simulink model "VehRT_211219"  (R2019b)
settings: Solver=ode5  StartTime=0.0  StopTime=Inf  FixedStep=Ts  RelTol=1e-3  EnableMultiTasking=on
InitFcn:
  | VehRT_Init_211219;
  | Ts=0.0005;
values from neighbouring files (symbols this model uses):
  damping_p = 0.113    [VehRT_Init_211219.m]
  Ff_ab_p = 0.41    [VehRT_Init_211219.m]
  Ff_c_p = 0.4    [VehRT_Init_211219.m]
  friction_enable = 1    [VehRT_Init_211219.m]
  sigma0_p = 200    [VehRT_Init_211219.m]
  sigma1_p = (200)^0.5    (= 14.1421356237)    [VehRT_Init_211219.m]
  td = 0.01    [VehRT_Init_211219.m]
  theta_sb_p = 0.03    [VehRT_Init_211219.m]
undefined symbols (not defined in the file or in its folder): C, canChannel, D, DiscIntNeverNeededParam, g, IO306, Kf, Kr, Lf, Lr, M, magnitude, sigma, trajectory_x11_, trajectory_x12_, trajectory_x13_, trajectory_x14_, trajectory_x15_, trajectory_x16_, trajectory_x17_, trajectory_x21_, trajectory_x22_, trajectory_x23_, trajectory_x24_, trajectory_x25_, trajectory_x26_, trajectory_x27_, trajectory_y11_, trajectory_y12_, trajectory_y13_, trajectory_y14_, trajectory_y15_, trajectory_y16_, trajectory_y17_, trajectory_y21_, trajectory_y22_, trajectory_y23_, trajectory_y24_, trajectory_y25_, trajectory_y26_, trajectory_y27_, zeta
libraries: canmsglib x31, speedgoatlib_IO612 x20, slrtlib x15, simulink x5, speedgoatlib_IO133 x3, xpcutilitieslib x2, canlib x2, xpcrtudplib x2, speedgoatlib_fpga x1, speedgoatlib_fpga_dio x1, autolibshared x1, speedgoatlib_fpga_quadrature x1
(part 2 of 4)

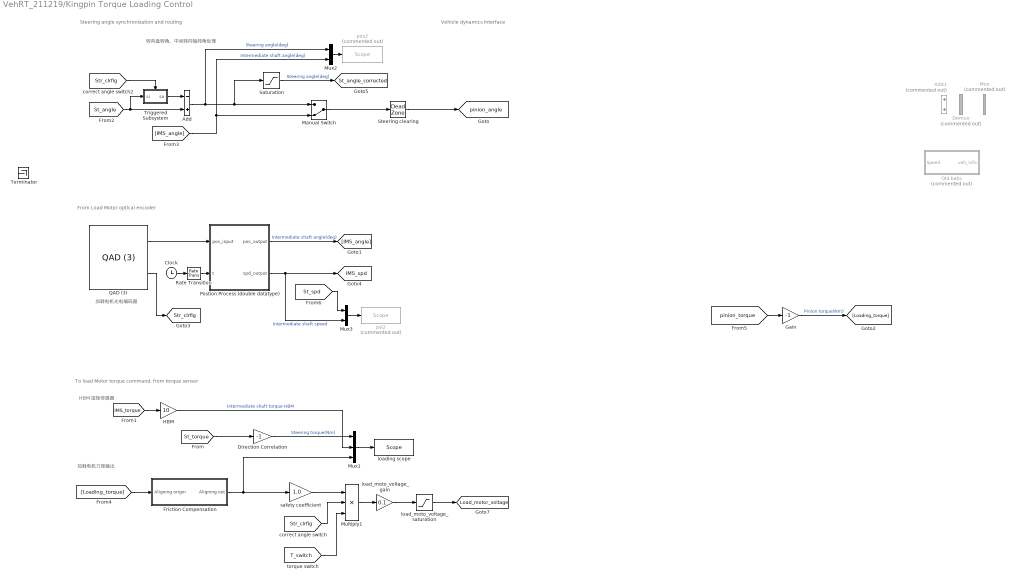
== system VehRT_211219/Kingpin Torque Loading Control ==
  note: To load Motor torque command, from torque sensor
  note: From Load Motor optical encoder
  note: Vehicle dynamics Interface
  note: Steering angle synchronization and routing
  note: 加载电机力矩输出
  note: 加载电机光电编码器
  note: HBM 扭矩传感器
  note: 转向盘转角、中间转向轴转角处理
  Add : Sum  Inputs=-+
  Add1 : Sum  Commented=on
  Clock : Clock
  Demux : Demux  Commented=on  Outputs=2
  Direction Correlation : Gain  Gain=-1
  Friction Compensation : Subsystem
  Gain : Gain  Gain=-1
  HBM : Gain  Gain=10
  Manual Switch : ManualSwitch  CurrentSetting=0
  Multiply1 : Product  Inputs=3
  Mux : Mux  Commented=on  Inputs=2
  Mux1 : Mux  Inputs=3
  Mux2 : Mux  Inputs=2
  Mux3 : Mux  Inputs=2
  Old baks : Subsystem  Commented=on
  Postion Process (double datatype) : MATLAB Function  TreatAsAtomicUnit=on
  QAD (3) : speedgoatlib_fpga_quadrature/QAD (3)  id=1  board=IO306-25k  chan=[1]  resetOnStart=on  ts=Ts  pciSlot=-1  operatingMode=Quadrature decoder  indexControlMode=Reset on index  resolution=4x  stepsPerRevolution=[6815744/2]  latchMode=Disabled  interpolatePosition=off  invertAB=off  showClearPositionInput=off  showClearIndexFoundInput=off  showPositionOutput=on  showTurnOutput=off  showSpeedOutput=off  showDirectionOutput=off  showIndexFoundOutput=on
      settings: SourceProductName=Simulink Real-Time: Speedgoat I/O Driver Library
  Rate Transition : RateTransition  Deterministic=off
  Saturation : Saturate  UpperLimit=90  LowerLimit=-90
  Steering clearing : DeadZone  LowerValue=0  UpperValue=0  SaturateOnIntegerOverflow=on
  Terminator : Terminator
  Triggered Subsystem : Subsystem  TreatAsAtomicUnit=on
  load_moto_voltage_gain : Gain  Gain=0.1
  load_moto_voltage_saturation : Saturate  UpperLimit=2.5  LowerLimit=-2.5
  loading scope : slrtlib/Displays and Logging/Scope   scopeno=3  scopetype=Target  autostart=on  viewmode=Graphical rolling  formatstr='%15.6f'  grid=on  ylimits=[-20,20]  nosamples=1000  noprepostsamples=0  interleave=1  triggermode=FreeRun  triggersignal=1  trigsignalfromport=off  triggerlevel=0.0  triggerslope=Either  triggerscope=1  triggersample=0  filename=data.dat  mode=Lazy  writesize=512  autorestart=off  dynamicfilemode=off  maxwritefilesize=512*1024^2
  "pos2 " : slrtlib/Displays and Logging/Scope   Commented=on  scopeno=1  scopetype=Target  autostart=on  viewmode=Graphical rolling  formatstr='%15.6f'  grid=on  ylimits=[-60,60]  nosamples=1000  noprepostsamples=0  interleave=1  triggermode=FreeRun  triggersignal=1  trigsignalfromport=off  triggerlevel=0.0  triggerslope=Either  triggerscope=1  triggersample=0  filename=data.dat  mode=Lazy  writesize=512  autorestart=off  dynamicfilemode=off  maxwritefilesize=512*1024^2
  psi2 : slrtlib/Displays and Logging/Scope   Commented=on  scopeno=2  scopetype=Target  autostart=on  viewmode=Graphical rolling  formatstr='%15.6f'  grid=on  ylimits=[-100,100]  nosamples=1000  noprepostsamples=0  interleave=1  triggermode=FreeRun  triggersignal=1  trigsignalfromport=off  triggerlevel=0.0  triggerslope=Either  triggerscope=1  triggersample=0  filename=data.dat  mode=Lazy  writesize=512  autorestart=off  dynamicfilemode=off  maxwritefilesize=512*1024^2
  safety coefficient : Gain  Gain=1.0
  tag scope: IMS_spd=global, Load_motor_voltage=global, St_angle_corrected=global, Str_clrflg=global, pinion_angle=global
  wires:
  load_moto_voltage_gain/1 -> load_moto_voltage_saturation/1
  HBM/1 -> Mux1/2  "Intermediate shaft torque HBM"
  Gain/1 -> [Loading_torque]  "Pinion torque(Nm)"
  [IMS_torque] -> HBM/1
  Add/1 -> Manual Switch/1, Saturation/1, Mux2/1  "Steering angle(deg)"
  QAD (3)/1 -> Postion Process (double datatype)/1(pos_input)
  [IMS_angle] -> Manual Switch/2, Mux2/2  "Intermediate shaft angle(deg)"
  Postion Process (double datatype)/1(pos_output) -> [IMS_angle]  "Intermediate shaft angle(deg)"
  safety coefficient/1 -> Multiply1/1
  load_moto_voltage_saturation/1 -> [Load_motor_voltage]
  Mux1/1 -> loading scope/1
  Manual Switch/1 -> Steering clearing/1
  Clock/1 -> Rate Transition/1
  Rate Transition/1 -> Postion Process (double datatype)/2(t)
  QAD (3)/2 -> [Str_clrflg]
  Postion Process (double datatype)/2(spd_output) -> [IMS_spd], Mux3/2  "Intermediate shaft speed"
  Triggered Subsystem/1(so) -> Add/1
  [Str_clrflg] -> Triggered Subsystem/Trigger
  [St_angle] -> Add/2, Triggered Subsystem/1(si)
  [Str_clrflg] -> Multiply1/2
  Multiply1/1 -> load_moto_voltage_gain/1
  [T_switch] -> Multiply1/3
  Mux2/1 -> "pos2 "/1
  Mux3/1 -> psi2/1
  [St_spd] -> Mux3/1
  [St_torque] -> Direction Correlation/1
  Direction Correlation/1 -> Mux1/1  "Steering torque(Nm)"
  Friction Compensation/1(Aligning out) -> safety coefficient/1, Mux1/3
  [Loading_torque] -> Friction Compensation/1(Aligning origin)
  Saturation/1 -> [St_angle_corrected]  "Steering angle(deg)"
  Steering clearing/1 -> [pinion_angle]
  [pinion_torque] -> Gain/1

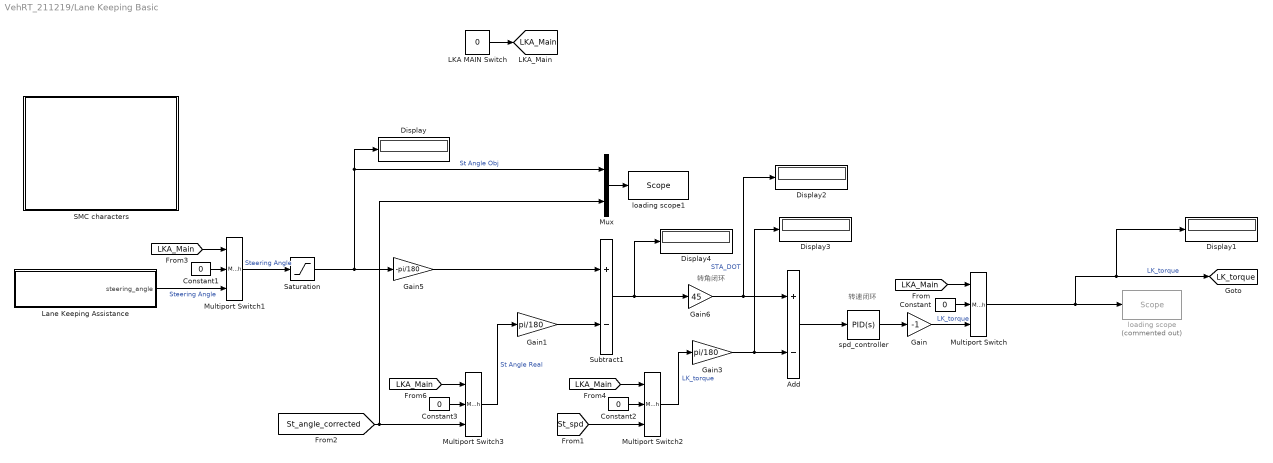
== system VehRT_211219/Lane Keeping Basic ==
  note: 转角闭环
  note: 转速闭环
  Add : Sum  Inputs=+-
  Constant{,1..3} (4 alike) : Constant  Value=0
  Display{,1..4} (5 alike) : Display
  Gain : Gain  Gain=-1
  Gain1 : Gain  Gain=pi/180
  Gain3 : Gain  Gain=pi/180
  Gain5 : Gain  Gain=-pi/180
  Gain6 : Gain  Gain=45
  LKA MAIN Switch : Constant  Value=0
  Lane Keeping Assistance : Subsystem
  Multiport Switch{,1..3} (4 alike) : MultiPortSwitch  DataPortOrder=Zero-based contiguous  Inputs=2  zeroidx=on
  Mux : Mux  Inputs=2
  SMC characters : Subsystem
  Saturation : Saturate  UpperLimit=70  LowerLimit=-70
  Subtract1 : Sum  Inputs=+-
  loading scope : slrtlib/Displays and Logging/Scope   Commented=on  scopeno=7  scopetype=Target  autostart=on  viewmode=Graphical rolling  formatstr='%15.6f'  grid=on  ylimits=[-2.5,2.5]  nosamples=1000  noprepostsamples=0  interleave=1  triggermode=FreeRun  triggersignal=1  trigsignalfromport=off  triggerlevel=0.0  triggerslope=Either  triggerscope=1  triggersample=0  filename=data.dat  mode=Lazy  writesize=512  autorestart=off  dynamicfilemode=off  maxwritefilesize=512*1024^2
  loading scope1 : slrtlib/Displays and Logging/Scope   scopeno=6  scopetype=Target  autostart=on  viewmode=Graphical rolling  formatstr='%15.6f'  grid=on  ylimits=[-50,50]  nosamples=1000  noprepostsamples=0  interleave=1  triggermode=FreeRun  triggersignal=1  trigsignalfromport=off  triggerlevel=0.0  triggerslope=Either  triggerscope=1  triggersample=0  filename=data.dat  mode=Lazy  writesize=512  autorestart=off  dynamicfilemode=off  maxwritefilesize=512*1024^2
  spd_controller : simulink/Continuous/PID Controller  Controller=PID  Form=Parallel  TimeDomain=Continuous-time  SampleTime=-1  IntegratorMethod=Forward Euler  FilterMethod=Forward Euler  ControllerParametersSource=internal  P=4.3  I=0  D=0.03  UseFilter=on  N=100  TunerSelectOption=Transfer Function Based (PID Tuner App)  InitialConditionSource=internal  InitialConditionForIntegrator=0  InitialConditionForFilter=0  DifferentiatorICPrevScaledInput=0  ExternalReset=none  TrackingMode=off  Kt=1  LimitOutput=on  UpperSaturationLimit=7  LowerSaturationLimit=-7  LinearizeAsGain=off  AntiWindupMode=none  Kb=1  POutMin=[]  POutMax=[]  IOutMin=[]  IOutMax=[]  DOutMin=[]  DOutMax=[]  NOutMin=[]  NOutMax=[]  SumOutMin=[]  SumOutMax=[]  SaturationOutMin=[]  SaturationOutMax=[]  PParamMin=[]  PParamMax=[]  IParamMin=[]  IParamMax=[]  DParamMin=[]  DParamMax=[]  NParamMin=[]  NParamMax=[]  KbParamMin=[]  KbParamMax=[]  KtParamMin=[]  KtParamMax=[]  KbOutMin=[]  KbOutMax=[]  KtOutMin=[]  KtOutMax=[]  IntegratorOutMin=[]  IntegratorOutMax=[]  FilterOutMin=[]  FilterOutMax=[]  SumI1OutMin=[]  SumI1OutMax=[]  SumI2OutMin=[]  SumI2OutMax=[]  SumI3OutMin=[]  SumI3OutMax=[]  SumI4OutMin=[]  SumI4OutMax=[]  SumDOutMin=[]  SumDOutMax=[]  DifferentiatorOutMin=[]  DifferentiatorOutMax=[]  FilterDiffOutCoefMin=[]  FilterDiffOutCoefMax=[]  ReciprocalOutMin=[]  ReciprocalOutMax=[]  SumDenOutMin=[]  SumDenOutMax=[]  SumNumOutMin=[]  SumNumOutMax=[]  DivideOutMin=[]  DivideOutMax=[]  IntegratorContinuousStateAttributes=''  IntegratorStateMustResolveToSignalObject=off  IntegratorRTWStateStorageClass=Auto  FilterContinuousStateAttributes=''  FilterStateMustResolveToSignalObject=off  FilterRTWStateStorageClass=Auto  ParallelPVariant=InternalParameters  IdealPVariant=Disabled  IVariant=InternalParameters  DVariant=InternalParameters  IntegratorVariant=Continuous  SatVariant=Enabled  AWVariant=Passthrough  PCopyVariant=Disabled  TRVariant=Disabled  FdbkBlocksVariant=Forward  IdealPFdbkVariant=Disabled  SatFdbkVariant=Disabled  DerivativeFilterVariant=ContFilter  NVariant=InternalParameters  NCopyVariant=Disabled  FilterICVariant=InternalICsFilter  IntegratorICVariant=InternalICs  ExternalResetVariant=Disabled  TRSumVariant=Passthrough  SumFdbkVariant=Disabled  SumVariant=Sum_PID
  tag scope: LKA_Main=global, LK_torque=global
  wires:
  Subtract1/1 -> Gain6/1, Display4/1
  Multiport Switch3/1 -> Gain1/1  "St Angle Real"
  Gain1/1 -> Subtract1/2
  Gain6/1 -> Display2/1, Add/1  "STA_DOT"
  Multiport Switch/1 -> loading scope/1, Display1/1, [LK_torque]  "LK_torque"
  [St_spd] -> Multiport Switch2/3
  Gain3/1 -> Display3/1, Add/2
  Add/1 -> spd_controller/1
  Mux/1 -> loading scope1/1
  spd_controller/1 -> Gain/1
  Saturation/1 -> Gain5/1, Mux/1, Display/1  "St Angle Obj"
  Multiport Switch1/1 -> Saturation/1  "Steering Angle"
  Gain5/1 -> Subtract1/1
  LKA MAIN Switch/1 -> [LKA_Main]
  [LKA_Main] -> Multiport Switch/1
  Constant/1 -> Multiport Switch/2
  Gain/1 -> Multiport Switch/3  "LK_torque"
  Constant1/1 -> Multiport Switch1/2
  [LKA_Main] -> Multiport Switch1/1
  Lane Keeping Assistance/1(steering_angle) -> Multiport Switch1/3  "Steering Angle"
  Constant2/1 -> Multiport Switch2/2
  [LKA_Main] -> Multiport Switch2/1
  Multiport Switch2/1 -> Gain3/1  "LK_torque"
  [LKA_Main] -> Multiport Switch3/1
  Constant3/1 -> Multiport Switch3/2
  [St_angle_corrected] -> Multiport Switch3/3, Mux/2

== system VehRT_211219/Vehicle Info ==
  Bus Selector : BusSelector  OutputSignals=drv_sta,drv_thr,drv_brk
  "Scope " : slrtlib/Displays and Logging/Scope   scopeno=112  scopetype=Target  autostart=on  viewmode=Graphical rolling  formatstr='%15.6f'  grid=on  ylimits=[0,1]  nosamples=8000  noprepostsamples=0  interleave=1  triggermode=FreeRun  triggersignal=1  trigsignalfromport=off  triggerlevel=0.0  triggerslope=Either  triggerscope=1  triggersample=0  filename=data.dat  mode=Lazy  writesize=512  autorestart=off  dynamicfilemode=off  maxwritefilesize=512*1024^2
  Scope 1 : slrtlib/Displays and Logging/Scope   scopeno=113  scopetype=Target  autostart=on  viewmode=Graphical rolling  formatstr='%15.6f'  grid=on  ylimits=[0,1]  nosamples=8000  noprepostsamples=0  interleave=1  triggermode=FreeRun  triggersignal=1  trigsignalfromport=off  triggerlevel=0.0  triggerslope=Either  triggerscope=1  triggersample=0  filename=data.dat  mode=Lazy  writesize=512  autorestart=off  dynamicfilemode=off  maxwritefilesize=512*1024^2
  Scope 2 : slrtlib/Displays and Logging/Scope   scopeno=111  scopetype=Target  autostart=on  viewmode=Graphical rolling  formatstr='%15.6f'  grid=on  ylimits=[-60,60]  nosamples=8000  noprepostsamples=0  interleave=1  triggermode=FreeRun  triggersignal=1  trigsignalfromport=off  triggerlevel=0.0  triggerslope=Either  triggerscope=1  triggersample=0  filename=data.dat  mode=Lazy  writesize=512  autorestart=off  dynamicfilemode=off  maxwritefilesize=512*1024^2
  drv_brk : Gain
  drv_sta : Gain
  drv_thr : Gain
  wires:
  [Veh_info] -> Bus Selector/1
  Bus Selector/1 -> drv_sta/1  "<drv_sta>"
  Bus Selector/2 -> drv_thr/1  "<drv_thr>"
  Bus Selector/3 -> drv_brk/1  "<drv_brk>"
  drv_thr/1 -> "Scope "/1  "drv_thr"
  drv_brk/1 -> Scope 1/1  "drv_brk"
  drv_sta/1 -> Scope 2/1  "drv_sta"

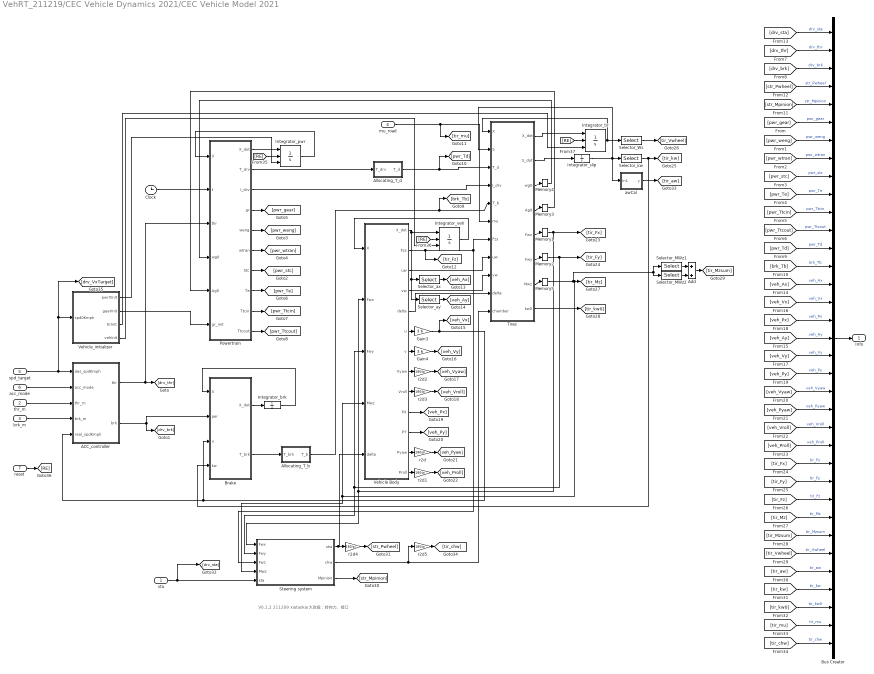
== system VehRT_211219/CEC Vehicle Dynamics 2021/CEC Vehicle Model 2021 ==
  note: V0.1.2 211209 xiataokai 大改版：转向力、接口
  sta : Inport
  thr_m : Inport  Port=2
  brk_m : Inport  Port=3
  mu_road : Inport  Port=4
  spd_target : Inport  Port=5
  acc_mode : Inport  Port=6
  reset : Inport  Port=7
  ACC_controller : Subsystem
  Add : Sum
  Allocating_T_b : Subsystem
  Allocating_T_d : Subsystem
  Brake : MATLAB Function
  Bus Creator : BusCreator  Inputs=35
  Clock : Clock
  Gain3 : Gain  Gain=3.6
  Gain4 : Gain  Gain=3.6
  Integrator_brk : Integrator  InitialCondition=zeros(5,1)  LimitOutput=on  UpperSaturationLimit=[1e9;1e9;1e9;1e9;1e9]  LowerSaturationLimit=[-1e9;-1e9;-1e9;-1e9;-1e9]
  Integrator_pwr : Integrator  ExternalReset=rising  InitialConditionSource=external  InitialCondition=[750/60*2*pi;0;0]  LimitOutput=on  UpperSaturationLimit=[1e9;1e9;1e9]  LowerSaturationLimit=[-1e9;-1e9;-1e9]
  Integrator_slip : Integrator  InitialCondition=zeros(8,1)  LimitOutput=on  UpperSaturationLimit=[1e9;1e9;1e9;1e9;1e9;1e9;1e9;1e9]  LowerSaturationLimit=[-1e9;-1e9;-1e9;-1e9;-1e9;-1e9;-1e9;-1e9]
  Integrator_tir : Integrator  ExternalReset=rising  InitialConditionSource=external  InitialCondition=zeros(6,1)  LimitOutput=on  UpperSaturationLimit=[1e9;1e9;1e9;1e9;1e9;1e9]  LowerSaturationLimit=[0;0;0;0;-1e9;-1e9]
  Integrator_veh : Integrator  ExternalReset=rising  InitialConditionSource=external  InitialCondition=zeros(8,1)  LimitOutput=on  UpperSaturationLimit=[1e9;1e9;1e9;1e9;1e9;1e9;1e9;1e9]  LowerSaturationLimit=[-1e9;-1e9; 0;-1e9;-1e9;-1e9;-1e9;-1e9]
  Memory{1..5} (5 alike) : Memory
  Powertrain : MATLAB Function
  Selector_MWz1 : Selector  InputPortWidth=4  IndexOptions=Index vector (dialog)  Indices=[1]  OutputSizes=1
  Selector_MWz2 : Selector  InputPortWidth=4  IndexOptions=Index vector (dialog)  Indices=[2]  OutputSizes=1
  Selector_Ws : Selector  InputPortWidth=6  IndexOptions=Index vector (dialog)  Indices=[1:4]  OutputSizes=1
  Selector_ax : Selector  InputPortWidth=8  IndexOptions=Index vector (dialog)  Indices=[3]  OutputSizes=1
  Selector_ay : Selector  InputPortWidth=8  IndexOptions=Index vector (dialog)  Indices=[4]  OutputSizes=1
  Selector_kw : Selector  InputPortWidth=8  IndexOptions=Index vector (dialog)  Indices=[1:4]  OutputSizes=1
  Steering system : Subsystem
  Tires : MATLAB Function  SystemSampleTime=0.001
  Vehicle Body : MATLAB Function  TreatAsAtomicUnit=on
      settings: MinAlgLoopOccurrences=on
  Vehicle_initializer : Subsystem
  awCal : Subsystem
  r2d{,1..5} (6 alike) : Gain  Gain=180/pi
  Info : Outport  VectorParamsAs1DForOutWhenUnconnected=off
  wires:
  Vehicle Body/12(Pyaw) -> r2d/1
  Vehicle_initializer/2(gearInit) -> Powertrain/6(gr_init)
  Tires/7(Mwz) -> Memory5/1
  Vehicle_initializer/1(pwrXInit) -> Integrator_pwr/3
  Vehicle_initializer/4(vehInit) -> Integrator_veh/3
  Memory2/1 -> [tir_Fy], Steering system/2(Fwy), Vehicle Body/3(Fwy)
  Powertrain/7(Stc) -> [pwr_stc]
  [RE] -> Integrator_veh/2
  [RE] -> Integrator_tir/2
  spd_target/1 -> [drv_VxTarget], Vehicle_initializer/1(spd0Kmph), ACC_controller/1(des_spdKmph)
  Selector_ax/1 -> [veh_Ax]
  Add/1 -> [tir_Mzsum]
  Clock/1 -> Powertrain/2(t)
  Integrator_pwr/1 -> Powertrain/1(X)
  Vehicle Body/4(vw) -> Tires/9(vw)
  Integrator_brk/1 -> Brake/1(X)
  Powertrain/2(T_drv) -> Allocating_T_d/1(T_drv)
  Gain3/1 -> [veh_Vx], ACC_controller/5(real_spdKmph), Brake/3(u)
  Brake/1(X_dot) -> Integrator_brk/1
  Brake/2(T_brk) -> Allocating_T_b/1(T_brk)
  Tires/6(Fwy) -> Memory2/1
  r2d3/1 -> [veh_Vroll]
  Gain4/1 -> [veh_Vy]
  Powertrain/6(wtran) -> [pwr_wtran]
  r2d2/1 -> [veh_Vyaw]
  Vehicle Body/6(u) -> Gain3/1
  Powertrain/5(weng) -> [pwr_weng]
  Allocating_T_d/1(T_d) -> [pwr_Td], Tires/3(T_d)
  ACC_controller/1(thr) -> Powertrain/3(thr), [drv_thr]
  Tires/2(S_dot) -> Integrator_slip/1
  Vehicle Body/3(uw) -> Tires/8(uw)
  [RE] -> Integrator_pwr/2
  Integrator_veh/1 -> Vehicle Body/1(X)
  Selector_ay/1 -> [veh_Ay]
  Vehicle Body/7(v) -> Gain4/1
  Tires/5(Fwx) -> Memory1/1
  Powertrain/3(I_drv) -> Tires/4(I_drv)
  Memory3/1 -> Powertrain/5(Ag0)
  Vehicle Body/5(delta) -> Tires/10(delta)
  Selector_MWz2/1 -> Add/2
  Powertrain/1(X_dot) -> Integrator_pwr/1
  mu_road/1 -> [tir_mu], Tires/6(mu)
  r2d1/1 -> [veh_Proll]
  Tires/3(wg0) -> Memory4/1
  Tires/4(Ag0) -> Memory3/1
  Selector_MWz1/1 -> Add/1
  ACC_controller/2(brk) -> Brake/2(per), [drv_brk]
  Vehicle Body/8(Vyaw) -> r2d2/1
  Integrator_slip/1 -> awCal/1(In1), Tires/2(S), Selector_kw/1
  Powertrain/4(gr) -> [pwr_gear]
  Selector_Ws/1 -> [tir_Vwheel]
  Integrator_tir/1 -> Tires/1(X), Selector_Ws/1
  Vehicle_initializer/3(tirInit) -> Integrator_tir/3
  Vehicle Body/9(Vroll) -> r2d3/1
  Vehicle Body/13(Proll) -> r2d1/1
  Memory4/1 -> Powertrain/4(wg0)
  Vehicle Body/1(X_dot) -> Selector_ax/1, Selector_ay/1, Integrator_veh/1
  Memory1/1 -> [tir_Fx], Steering system/1(Fwx), Vehicle Body/2(Fwx)
  Vehicle Body/2(Fzs) -> [tir_Fz], Steering system/3(Fwz), Tires/7(Fzs)
  Allocating_T_b/1(T_b) -> [brk_Tb], Tires/5(T_b)
  Selector_kw/1 -> [tir_kw], Brake/4(kw)
  Tires/1(X_dot) -> Integrator_tir/1
  r2d/1 -> [veh_Pyaw]
  Tires/8(kw0) -> [tir_kw0]
  Memory5/1 -> [tir_Mz], Steering system/4(Mwz), Vehicle Body/4(Mwz), Selector_MWz2/1, Selector_MWz1/1
  sta/1 -> [drv_sta], Steering system/5(sta)
  Steering system/1(stw) -> Vehicle Body/5("delta "), r2d4/1
  Steering system/3(Mpinion) -> [str_Mpinion]
  Steering system/2(chw) -> Tires/11(chamber), r2d5/1
  Vehicle Body/10(PX) -> [veh_Px]
  Vehicle Body/11(PY) -> [veh_Py]
  Powertrain/8(Te) -> [pwr_Te]
  Powertrain/9(Ttcin) -> [pwr_Ttcin]
  Powertrain/10(Ttcout) -> [pwr_Ttcout]
  r2d4/1 -> [str_Pwheel]
  awCal/1(y) -> [tir_aw]
  [drv_sta] -> Bus Creator/1  "drv_sta"
  [drv_thr] -> Bus Creator/2  "drv_thr"
  [drv_brk] -> Bus Creator/3  "drv_brk"
  [str_Pwheel] -> Bus Creator/4  "str_Pwheel"
  [str_Mpinion] -> Bus Creator/5  "str_Mpinion"
  [pwr_gear] -> Bus Creator/6  "pwr_gear"
  [pwr_weng] -> Bus Creator/7  "pwr_weng"
  [pwr_wtran] -> Bus Creator/8  "pwr_wtran"
  [pwr_stc] -> Bus Creator/9  "pwr_stc"
  [pwr_Te] -> Bus Creator/10  "pwr_Te"
  [pwr_Ttcin] -> Bus Creator/11  "pwr_Ttcin"
  [pwr_Ttcout] -> Bus Creator/12  "pwr_Ttcout"
  [pwr_Td] -> Bus Creator/13  "pwr_Td"
  [brk_Tb] -> Bus Creator/14  "brk_Tb"
  [veh_Ax] -> Bus Creator/15  "veh_Ax"
  [veh_Vx] -> Bus Creator/16  "veh_Vx"
  [veh_Px] -> Bus Creator/17  "veh_Px"
  [veh_Ay] -> Bus Creator/18  "veh_Ay"
  [veh_Vy] -> Bus Creator/19  "veh_Vy"
  [veh_Py] -> Bus Creator/20  "veh_Py"
  [veh_Vyaw] -> Bus Creator/21  "veh_Vyaw"
  [veh_Pyaw] -> Bus Creator/22  "veh_Pyaw"
  [veh_Vroll] -> Bus Creator/23  "veh_Vroll"
  [veh_Proll] -> Bus Creator/24  "veh_Proll"
  [tir_Fx] -> Bus Creator/25  "tir_Fx"
  [tir_Fy] -> Bus Creator/26  "tir_Fy"
  [tir_Fz] -> Bus Creator/27  "tir_Fz"
  [tir_Mz] -> Bus Creator/28  "tir_Mz"
  [tir_Mzsum] -> Bus Creator/29  "tir_Mzsum"
  [tir_Vwheel] -> Bus Creator/30  "tir_Vwheel"
  [tir_aw] -> Bus Creator/31  "tir_aw"
  [tir_kw] -> Bus Creator/32  "tir_kw"
  [tir_kw0] -> Bus Creator/33  "tir_kw0"
  [tir_mu] -> Bus Creator/34  "tir_mu"
  [tir_chw] -> Bus Creator/35  "tir_chw"
  r2d5/1 -> [tir_chw]
  Bus Creator/1 -> Info/1
  acc_mode/1 -> ACC_controller/2(acc_mode)
  thr_m/1 -> ACC_controller/3(thr_m)
  brk_m/1 -> ACC_controller/4(brk_m)
  reset/1 -> [RE]

== system VehRT_211219/CEC Vehicle Dynamics 2021/Reset with Clutch ==
  Clock : Clock
  Reset Funvtion : MATLAB Function  TreatAsAtomicUnit=on  SystemSampleTime=0.001
  rst : Outport
  wires:
  Reset Funvtion/1(rst) -> rst/1
  Clock/1 -> Reset Funvtion/2(t)
  [pedal_clt] -> Reset Funvtion/1(clt)

== system VehRT_211219/CEC Vehicle Dynamics 2021/mu_test ==
  Manual Switch : ManualSwitch  CurrentSetting=0
  Vector Concatenate : Concatenate  NumInputs=4
  mu=0.85 : Constant  Value=ones(4,1)*0.85
  mu=1~0.2 : Step  Time=17.5  Before=1  After=0.2  SampleTime=0
  mu=1~0.2_2 : Step  Time=17.5  Before=1  After=0.2  SampleTime=0
  mu=1~0.2_3 : Step  Time=17.5  Before=1  After=0.2  SampleTime=0
  mu=1~0.2_4 : Step  Time=17.5  Before=1  After=0.2  SampleTime=0
  mus : Outport
  wires:
  mu=1~0.2_4/1 -> Vector Concatenate/4
  mu=1~0.2/1 -> Vector Concatenate/1
  mu=1~0.2_2/1 -> Vector Concatenate/2
  Vector Concatenate/1 -> Manual Switch/1
  mu=1~0.2_3/1 -> Vector Concatenate/3
  Manual Switch/1 -> mus/1
  mu=0.85/1 -> Manual Switch/2

== system VehRT_211219/Connect Scenery/Backup ==
  "Byte Packing " : xpcutilitieslib/Byte Packing   Commented=on  MaskPackedDataType=uint8  MaskUnpackedDataTypes={'double'}  MaskAlignment=1
  Byte Unpacking 1 : xpcutilitieslib/Byte Unpacking   Commented=on  MaskUnpackedDataTypes={'double'}  MaskUnpackedDataSizes={[2]}  MaskAlignment=1
      settings: SourceProductName=Simulink Real-Time  SourceProductBaseCode=XP
  CAN Configuration : canlib/CAN Configuration  Commented=on  BlockHandle=1343.0002  Device=MathWorks Virtual 1 (Channel 1)  DeviceMenu=MathWorks Virtual 1 (Channel 1)  ObjConstructor=canChannel('MathWorks', 'Virtual 1', 1)  BusSpeed=1000000  EnableBitParameters=off  SJW=1  TSEG1=4  TSEG2=3  NSamples=1  AckMode=Normal
      settings: SourceProductName=Vehicle Network Toolbox  SourceProductBaseCode=VN
  CAN Receive : canlib/CAN Receive  Commented=on  BlockHandle=1344.0002  Device=MathWorks Virtual 1 (Channel 1)  DeviceMenu=MathWorks Virtual 1 (Channel 1)  ObjConstructor=canChannel('MathWorks', 'Virtual 1', 1)  EnableStandardIDsFilter=off  StdIDsCombo=Allow all  StandardIDs=0  EnableExtendedIDsFilter=off  ExtIDsCombo=Allow all  ExtendedIDs=0  SampleTime=0.01  MsgsPerTimestep=all  InternalFilterUpdateStatus=on  BusOutput=off
      settings: SourceProductName=Vehicle Network Toolbox  SourceProductBaseCode=VN
  CAN Unpack : canmsglib/CAN Unpack  Commented=on  MsgList=(none)  MsgName=CAN Msg  MsgIDType=Standard (11-bit identifier)  MsgIdentifier=0  MsgLength=8  SignalInfo={}  IDPort=off  TimestampPort=off  ErrorPort=off  RemotePort=off  LengthPort=off  StatusPort=off  ApplyMinMax=off
      settings: SourceProductName=Vehicle Network Toolbox  SourceProductBaseCode=VN  DataFormat=raw data
  CAN Write{1..6} (6 alike) : speedgoatlib_IO612/CAN Write  id=1  sampleTime=0.005  portSelection=2  messageType=CAN  enaStatusPort=off  protl=IO612  ptIdx=1  isFDMod=0
      settings: SourceProductName=Simulink Real-Time: Speedgoat Library
  Demux1 : Demux  Commented=on  Outputs=2
  Display1 : Display  Commented=on
  From1 : From  Commented=on  GotoTag=pedal_acc  TagVisibility=global
  From4 : From  Commented=on  GotoTag=pedal_brk  TagVisibility=global
  Mux : Mux  Commented=on  Inputs=12
  Mux1 : Mux  Commented=on  Inputs=2
  Receive1 : xpcrtudplib/UDP Receive  Commented=on  ipAddressVal=Use host-target connection  localPort=22222  rcvWidth=16  rcvFmAny=off  fmAddress=192.168.7.23  rcvMulticast=off  multicastAddress=[]  maxUDPQueue=8  sampleTime=-1
      settings: SourceProductName=Simulink Real-Time
  Reference : Sin  Commented=on  SampleTime=0
  Reference2 : simulink/Sources/Repeating Sequence  Commented=on  rep_seq_t=[0 2]  rep_seq_y=[-2 2]
  Scope : Scope  Commented=on
  "Scope " : slrtlib/Displays and Logging/Scope   Commented=on  scopeno=1  scopetype=Target  autostart=on  viewmode=Graphical sliding  formatstr='%15.6f'  grid=on  ylimits=[-1,1]  nosamples=4000  noprepostsamples=0  interleave=1  triggermode=FreeRun  triggersignal=1  trigsignalfromport=off  triggerlevel=0.0  triggerslope=Either  triggerscope=1  triggersample=0  filename=data.dat  mode=Lazy  writesize=512  autorestart=off  dynamicfilemode=off  maxwritefilesize=512*1024^2
  Send1 : xpcrtudplib/UDP Send  Commented=on  ipAddressVal=Use host-target connection  localPort=-1  toAddress=192.168.7.23  toPort=1234  sampleTime=0.05
      settings: SourceProductName=Simulink Real-Time  SourceProductBaseCode=XP
  "Vxzb0 " : Gain  Commented=on
  Width : Width  Commented=on
  phi_Gain : Gain
  theta_Gain : Gain
  wires:
  ? -> Mux/11
  ? -> Mux/12
  Receive1/1 -> Byte Unpacking 1/1
  Mux/1 -> "Byte Packing "/1
  "Vxzb0 "/1 -> Scope/1
  From1/1 -> Mux/9
  Demux1/1 -> Mux1/2  "feedback"
  Byte Unpacking 1/1 -> Demux1/1  "feedback"
  Demux1/2 -> "Vxzb0 "/1
  Mux1/1 -> "Scope "/1
  Receive1/2 -> Display1/1
  Reference2/1 -> Mux/7, Mux1/1  "origin"
  "Byte Packing "/1 -> Width/1, Send1/1
  Width/1 -> Send1/2
  From4/1 -> Mux/10
  ? -> phi_Gain/1  "<phi>"
  ? -> theta_Gain/1  "<theta>"

== system VehRT_211219/Connect Scenery/CAN Receiver Port4 ==
  CAN Read1 : speedgoatlib_IO612/CAN Read  id=1  sampleTime=-1  portSelection=2  messageType=CAN  protl=IO612  ptIdx=1  isFDMod=0
      settings: SourceProductName=Simulink Real-Time: Speedgoat Library
  CAN Unpack : canmsglib/CAN Unpack  CANdbFile=D:\Speedgoat\Simulink Test Model\EPS_Test_2018_0101.dbc  MsgList=EPS2MAB  MsgName=CAN Msg  MsgIDType=Standard (11-bit identifier)  MsgIdentifier=500  MsgLength=8  SignalInfo={ 'Vx_des', '16', '32', 'LE', 'single', 'Standard', '0', '1', '0', '-Inf', 'Inf'; 'detection', '48', '16', 'LE', 'unsigned', 'Standard', '0', '1', '0', '-Inf', 'Inf'; 'road_id', '0', '16', 'LE', 'unsigned', 'Standard', '0', '1', '0', '-Inf', 'Inf' }  IDPort=off  TimestampPort=off  ErrorPort=off  RemotePort=off  LengthPort=off  StatusPort=off  ApplyMinMax=off
      settings: SourceProductName=Simulink Real-Time
  CAN Unpack1 : canmsglib/CAN Unpack  CANdbFile=D:\Speedgoat\Simulink Test Model\EPS_Test_2018_0101.dbc  MsgList=EPS2MAB  MsgName=VSS1  MsgIDType=Standard (11-bit identifier)  MsgIdentifier=501  MsgLength=8  SignalInfo={ 'range', '0', '64', 'LE', 'double', 'Standard', '0', '1', '0', '-Inf', 'Inf' }  IDPort=off  TimestampPort=off  ErrorPort=off  RemotePort=off  LengthPort=off  StatusPort=off  ApplyMinMax=off
      settings: SourceProductName=Simulink Real-Time
  CAN Unpack2 : canmsglib/CAN Unpack  CANdbFile=D:\Speedgoat\Simulink Test Model\EPS_Test_2018_0101.dbc  MsgList=EPS2MAB  MsgName=VSS2  MsgIDType=Standard (11-bit identifier)  MsgIdentifier=502  MsgLength=8  SignalInfo={ 'theta', '0', '64', 'LE', 'double', 'Standard', '0', '1', '0', '-Inf', 'Inf' }  IDPort=off  TimestampPort=off  ErrorPort=off  RemotePort=off  LengthPort=off  StatusPort=off  ApplyMinMax=off
      settings: SourceProductName=Simulink Real-Time
  CAN Unpack3 : canmsglib/CAN Unpack  CANdbFile=D:\Speedgoat\Simulink Test Model\EPS_Test_2018_0101.dbc  MsgList=EPS2MAB  MsgName=VSS3  MsgIDType=Standard (11-bit identifier)  MsgIdentifier=503  MsgLength=8  SignalInfo={ 'head_ada', '0', '64', 'LE', 'double', 'Standard', '0', '1', '0', '-Inf', 'Inf' }  IDPort=off  TimestampPort=off  ErrorPort=off  RemotePort=off  LengthPort=off  StatusPort=off  ApplyMinMax=off
      settings: SourceProductName=Simulink Real-Time
  While Iterator : WhileIterator  WhileBlockType=do-while
  detection : Outport
  Vx_des : Outport  Port=2
  devia_from_prescan : Outport  Port=3
  qulv_from_prescan : Outport  Port=4
  head_ada : Outport  Port=5
  road_id : Outport  Port=6
  wires:
  CAN Read1/1 -> While Iterator/1
  CAN Read1/2 -> CAN Unpack3/1, CAN Unpack2/1, CAN Unpack1/1, CAN Unpack/1
  CAN Unpack/1 -> Vx_des/1  "Vx_des"
  CAN Unpack/2 -> detection/1  "detection"
  CAN Unpack/3 -> road_id/1
  CAN Unpack1/1 -> devia_from_prescan/1  "range"
  CAN Unpack2/1 -> qulv_from_prescan/1  "theta"
  CAN Unpack3/1 -> head_ada/1  "head_ada"

== system VehRT_211219/EPS Steering Torque Assist Control/Backups ==
  note: 备用的滞后-超前控制
  note: 备用的超前控制
  Lag Control1 : TransferFcn  Commented=on  Numerator=[1/2/pi/4.5 1]  Denominator=[1/2/pi/1 1]
  Lead Control : TransferFcn  Commented=on  Numerator=[1/2/pi/14 1]  Denominator=[1/2/pi/181 1]
  Lead Control1 : TransferFcn  Commented=on  Numerator=[1/2/pi/14 1]  Denominator=[1/2/pi/100 1]
  Relay : Relay  Commented=on  OnSwitchValue=10  OffSwitchValue=-10
  Terminator : Terminator
  wires:
  Lag Control1/1 -> Lead Control1/1
  [Vehicle_speed] -> Terminator/1

== system VehRT_211219/Hardware Interfaces/RPM Display ==
  Bus Selector : BusSelector  OutputSignals=pwr_weng
  MATLAB Function : MATLAB Function  TreatAsAtomicUnit=on
  Out1 : Outport
  wires:
  [Veh_info] -> Bus Selector/1
  Bus Selector/1 -> MATLAB Function/1(rpm)  "<pwr_weng>"
  MATLAB Function/1(out) -> Out1/1

== system VehRT_211219/Hardware Interfaces/Shiftting Display ==
  Bus Selector : BusSelector  OutputSignals=pwr_gear
  MATLAB Function : MATLAB Function  TreatAsAtomicUnit=on
  Out1 : Outport
  wires:
  [Veh_info] -> Bus Selector/1
  Bus Selector/1 -> MATLAB Function/1(gear)  "<pwr_gear>"
  MATLAB Function/1(out) -> Out1/1

== system VehRT_211219/Hardware Interfaces/Spd Dev ==
  In1 : Inport
  Add : Sum
  Gain : Gain  Gain=0.5
  Memory : Memory
  Transfer Fcn : TransferFcn  Numerator=[100 0]  Denominator=[1 100]
  Out1 : Outport  VectorParamsAs1DForOutWhenUnconnected=off
  wires:
  In1/1 -> Transfer Fcn/1
  Transfer Fcn/1 -> Add/2, Memory/1
  Memory/1 -> Add/1
  Add/1 -> Gain/1
  Gain/1 -> Out1/1  "Steering speed(deg/s)"

== system VehRT_211219/Hardware Interfaces/Torque Switch Interface  ==
  b_on : Inport
  b_off : Inport  Port=2
  Constant1 : Constant  Value=9.9
  Multiport Switch : MultiPortSwitch  DataPortOrder=Zero-based contiguous  Inputs=2  zeroidx=on
  Sine Wave : Sin  Amplitude=6  Frequency=9  SampleTime=0
  torque switch : MATLAB Function  TreatAsAtomicUnit=on
  Out1 : Outport  VectorParamsAs1DForOutWhenUnconnected=off
  tag scope: T_switch=global
  wires:
  torque switch/1(control) -> [T_switch], Multiport Switch/1
  b_off/1 -> torque switch/2(button_off)  "b_off"
  Constant1/1 -> Multiport Switch/3
  Sine Wave/1 -> Multiport Switch/2
  Multiport Switch/1 -> Out1/1
  b_on/1 -> torque switch/1(button_on)  "b_on"

== system VehRT_211219/Hardware Interfaces/While Iterator Subsystem ==
  Add2 : Sum  Inputs=+-
  CAN Read1 : speedgoatlib_IO612/CAN Read  id=1  sampleTime=-1  portSelection=1  messageType=CAN  protl=IO612  ptIdx=0  isFDMod=0
      settings: SourceProductName=Simulink Real-Time: Speedgoat Library
  CAN Unpack : canmsglib/CAN Unpack  CANdbFile=D:\Speedgoat\Simulink Test Model\EPS_Test_2018_0101.dbc  MsgList=EPS2MAB  MsgName=EPS2MAB  MsgIDType=Standard (11-bit identifier)  MsgIdentifier=2043  MsgLength=8  SignalInfo={'MotorAngle','24','32','BE','signed','Standard','0','0.0043945','0','-Inf','Inf';'MotorCurrent','40','16','BE','signed','Standard','0','0.01','0','-Inf','Inf';'TorqueSensor','56','16','BE','signed','Standard','0','0.001','0','-Inf','Inf'}  IDPort=off  TimestampPort=on  ErrorPort=off  RemotePort=off  LengthPort=off  StatusPort=on  ApplyMinMax=off
      settings: SourceProductName=Simulink Real-Time  DataFormat=CANdb specified signals
  Demux : Demux  Commented=on  Outputs=3
  Gain3 : Gain  Gain=1/18.5
  Memory2 : Memory  InheritSampleTime=on
  Product : Product  Commented=on
  Saturation1 : Saturate  Commented=on  UpperLimit=120  LowerLimit=-120
  State-Space1 : StateSpace  Commented=on  A=[0,1,0; 0,0,1; -10/0.003^3,-10/0.003^2,-10/0.003]  B=[0;0;10/0.003^3]  C=[1,0,0;0,1,0;0,0,1]  D=[0;0;0]  InitialCondition=0
  Step : Step  Commented=on  Time=1.5  SampleTime=0
  Terminator{2..3,6,9} (4 alike) : Terminator
  Terminator4 : Terminator  Commented=on
  Terminator5 : Terminator  Commented=on
  While Iterator : WhileIterator  WhileBlockType=do-while
  st_angle : Outport  VectorParamsAs1DForOutWhenUnconnected=off
  st_torque : Outport  Port=2  VectorParamsAs1DForOutWhenUnconnected=off
  st_current : Outport  Port=3  VectorParamsAs1DForOutWhenUnconnected=off
  wires:
  CAN Unpack/2 -> st_current/1  "motor_current"
  Demux/1 -> Terminator5/1  "angle"
  CAN Read1/1 -> While Iterator/1
  CAN Read1/2 -> CAN Unpack/1
  CAN Unpack/4 -> Add2/1, Memory2/1  "TimeStamp"
  CAN Unpack/5 -> Terminator2/1
  Demux/2 -> Product/2
  Add2/1 -> Terminator3/1  "message_interval"
  Step/1 -> Product/1
  Memory2/1 -> Add2/2
  CAN Unpack/1 -> Gain3/1  "motor_angle"
  Gain3/1 -> st_angle/1, State-Space1/1  "Steering wheel angle0"
  CAN Unpack/3 -> Terminator6/1, st_torque/1  "Steering wheel torque"
  Product/1 -> Saturation1/1
  Saturation1/1 -> Terminator9/1
  State-Space1/1 -> Demux/1
  Demux/3 -> Terminator4/1  "acceleration"

== system VehRT_211219/Hardware Interfaces/alpha_dis ==
  CAN Read1 : speedgoatlib_IO612/CAN Read  id=1  sampleTime=-1  portSelection=2  messageType=CAN  protl=IO612  ptIdx=1  isFDMod=0
      settings: SourceProductName=Simulink Real-Time: Speedgoat Library
  CAN Unpack : canmsglib/CAN Unpack  CANdbFile=D:\Speedgoat\Simulink Test Model\EPS_Test_2018_0101.dbc  MsgList=EPS2MAB  MsgName=ALPHA  MsgIDType=Standard (11-bit identifier)  MsgIdentifier=450  MsgLength=8  SignalInfo={'alpha','0','32','LE','single','Standard','0','1','0','-Inf','Inf'}  IDPort=off  TimestampPort=off  ErrorPort=off  RemotePort=off  LengthPort=off  StatusPort=off  ApplyMinMax=off
      settings: SourceProductName=Simulink Real-Time
  Data Type Conversion1 : DataTypeConversion  OutMin=0  OutMax=8  OutDataTypeStr=uint16  RndMeth=Nearest
  Gain : Gain  Gain=8.5
  Saturation : Saturate  UpperLimit=8.5  LowerLimit=0
  While Iterator : WhileIterator  WhileBlockType=do-while
  alpha : Outport  VectorParamsAs1DForOutWhenUnconnected=off
  wires:
  CAN Read1/1 -> While Iterator/1
  CAN Read1/2 -> CAN Unpack/1
  CAN Unpack/1 -> Gain/1  "alpha"
  Gain/1 -> Saturation/1
  Saturation/1 -> Data Type Conversion1/1
  Data Type Conversion1/1 -> alpha/1

== system VehRT_211219/Kingpin Torque Loading Control/Friction Compensation ==
  note: 加上以后会抖，而且不怎么影响手感，所以暂时不加了
  note: 摩擦补偿
  note: 阻尼补偿
  Aligning origin : Inport
  Add : Sum
  Add1 : Sum
  DAM Friction_p : Subsystem
  Damping coefficient : Gain  Gain=damping_p
  Dead Zone : DeadZone  LowerValue=-0.15  UpperValue=0.15  SaturateOnIntegerOverflow=on
  Deg2Rad : Gain  Gain=-pi/180
  Fricompmode : Constant
  Low Pass Filter : TransferFcn  Denominator=[1/2/pi/20 1]
  Multiport Switch : MultiPortSwitch  DataPortOrder=Zero-based contiguous  Inputs=2  zeroidx=on
  Aligning out : Outport  VectorParamsAs1DForOutWhenUnconnected=off
  wires:
  Aligning origin/1 -> Multiport Switch/2, Add/1
  [IMS_spd] -> Deg2Rad/1
  Deg2Rad/1 -> Dead Zone/1, DAM Friction_p/1(velocity)
  Damping coefficient/1 -> Add1/2
  Dead Zone/1 -> Damping coefficient/1
  Add/1 -> Multiport Switch/3  "Aligning torque(Nm)"
  Multiport Switch/1 -> Aligning out/1  "Aligning torque"
  Fricompmode/1 -> Multiport Switch/1
  Add1/1 -> Low Pass Filter/1
  DAM Friction_p/1(friction) -> Add1/1
  Low Pass Filter/1 -> Add/2

== system VehRT_211219/Kingpin Torque Loading Control/Old baks ==
  note: SIMULINK三自由度车辆模型
  Speed : Inport
  1DLT_SpdPrtc : Lookup_n-D  NumberOfTableDimensions=1  BreakpointsForDimension1=[0 3 8 200]  Table=[0 0 1 1]  InternalRulePriority=Speed  RndMeth=Simplest  InputSameDT=on
  Aligning Torque Calculator : Subsystem
  Divide1 : Product  Inputs=/*
  Gain : Gain  Gain=1/3.6
  Gain2 : Gain  Gain=pi/180
  Multiply : Product
  Multiply2 : Product
  Terminator2 : Terminator
  Terminator3 : Terminator
  Trigonometric Function1 : Trigonometry  Operator=atan
  Vehicle Body 3DOF Single Track1 : autolibshared/Vehicle Body 3DOF Single Track  trackMode=Single (bicycle)  inputMode=External longitudinal velocity  frontSteerMode=on  rearSteerMode=off  windMode=off  muMode=off  extFMode=off  extMMode=off  extXo=off  extpsio=off  extxdoto=off  extro=off  extYo=off  extTamb=off  extydoto=off  aMode=2  NF=2  NR=2  m=M  a=Lf  b=Lr  h=0.35  X_o=0  xdot_o=0  CalphaMode=off  sigmaMode=off  d=0  w=[1.4,1.4]  Cy_f=Kf*2  Cy_r=Kr*2  sigma_f=.1  sigma_r=.1  alpha_f_brk=[-.1 .1]  Cy_f_data=[-9e3 9e3]  alpha_r_brk=[-.1 .1]  Cy_r_data=[-9e3 9e3]  Y_o=0  ydot_o=0  Izz=I  psi_o=0  r_o=0  Af=0  Cd=.3  Cl=.1  Cpm=.1  beta_w=[0:0.01:0.3]  Cs=[0:0.03:0.9]  Cym=[0:0.01:0.3]  Pabs=101325  Tair=273  g=g  mu=1  xdot_tol=.01  Fznom=5000  Fxtire_sat=7e4  Fytire_sat=7e4  longOff=0  latOff=0  vertOff=0  wrapAng=off
      settings: SourceProductName=Powertrain Blockset  SourceProductBaseCode=PW
  Yaw Gain : Gain
  angle_saturation_rad1 : Saturate  UpperLimit=1.5  LowerLimit=-1.5
  veh_info : Outport  VectorParamsAs1DForOutWhenUnconnected=off
  tag scope: Veh_info=global
  wires:
  Vehicle Body 3DOF Single Track1/6 -> Aligning Torque Calculator/3(Fzf)  "Fzf"
  Aligning Torque Calculator/1(Tire Aligning Torque) -> Multiply2/1
  angle_saturation_rad1/1 -> Vehicle Body 3DOF Single Track1/1, Aligning Torque Calculator/5(Delta)
  Multiply/1 -> Gain/1
  Vehicle Body 3DOF Single Track1/4 -> Terminator2/1  "psi"
  Vehicle Body 3DOF Single Track1/5 -> Yaw Gain/1  "r"
  1DLT_SpdPrtc/1 -> Multiply2/2
  Multiply2/1 -> ?
  Speed/1 -> 1DLT_SpdPrtc/1, Multiply/1
  [Str_clrflg] -> Multiply/2
  Vehicle Body 3DOF Single Track1/2 -> Divide1/1  "xdot"
  Vehicle Body 3DOF Single Track1/1 -> [Veh_info], veh_info/1
  Trigonometric Function1/1 -> Aligning Torque Calculator/1(Beta)  "Beta"
  Vehicle Body 3DOF Single Track1/7 -> Terminator3/1
  Vehicle Body 3DOF Single Track1/3 -> Divide1/2  "ydot"
  Gain/1 -> Vehicle Body 3DOF Single Track1/2, Aligning Torque Calculator/4(speed)
  Yaw Gain/1 -> Aligning Torque Calculator/2(r)  "r"
  Gain2/1 -> angle_saturation_rad1/1
  ? -> Gain2/1
  Divide1/1 -> Trigonometric Function1/1

== system VehRT_211219/Kingpin Torque Loading Control/Triggered Subsystem ==
  si : Inport
  Trigger : TriggerPort  VariantControl=Variant
  so : Outport  VectorParamsAs1DForOutWhenUnconnected=off
  wires:
  si/1 -> so/1

== system VehRT_211219/Lane Keeping Basic/Lane Keeping Assistance ==
  Constant : Constant  Value=0
  Constant1 : Constant  Value=0
  Constant2 : Constant  Value=0
  Multiport Switch : MultiPortSwitch  DataPortOrder=Zero-based contiguous  Inputs=2  zeroidx=on
  Multiport Switch1 : MultiPortSwitch  DataPortOrder=Zero-based contiguous  Inputs=2  zeroidx=on
  Multiport Switch2 : MultiPortSwitch  DataPortOrder=Zero-based contiguous  Inputs=2  zeroidx=on
  PID Controller : simulink/Continuous/PID Controller  Controller=PID  Form=Parallel  TimeDomain=Continuous-time  SampleTime=-1  IntegratorMethod=Forward Euler  FilterMethod=Forward Euler  ControllerParametersSource=internal  P=20  I=0  D=0  UseFilter=on  N=100  TunerSelectOption=Transfer Function Based (PID Tuner App)  InitialConditionSource=internal  InitialConditionForIntegrator=0  InitialConditionForFilter=0  DifferentiatorICPrevScaledInput=0  ExternalReset=none  TrackingMode=off  Kt=1  LimitOutput=off  UpperSaturationLimit=inf  LowerSaturationLimit=-inf  LinearizeAsGain=on  AntiWindupMode=none  Kb=1  POutMin=[]  POutMax=[]  IOutMin=[]  IOutMax=[]  DOutMin=[]  DOutMax=[]  NOutMin=[]  NOutMax=[]  SumOutMin=[]  SumOutMax=[]  SaturationOutMin=[]  SaturationOutMax=[]  PParamMin=[]  PParamMax=[]  IParamMin=[]  IParamMax=[]  DParamMin=[]  DParamMax=[]  NParamMin=[]  NParamMax=[]  KbParamMin=[]  KbParamMax=[]  KtParamMin=[]  KtParamMax=[]  KbOutMin=[]  KbOutMax=[]  KtOutMin=[]  KtOutMax=[]  IntegratorOutMin=[]  IntegratorOutMax=[]  FilterOutMin=[]  FilterOutMax=[]  SumI1OutMin=[]  SumI1OutMax=[]  SumI2OutMin=[]  SumI2OutMax=[]  SumI3OutMin=[]  SumI3OutMax=[]  SumI4OutMin=[]  SumI4OutMax=[]  SumDOutMin=[]  SumDOutMax=[]  DifferentiatorOutMin=[]  DifferentiatorOutMax=[]  FilterDiffOutCoefMin=[]  FilterDiffOutCoefMax=[]  ReciprocalOutMin=[]  ReciprocalOutMax=[]  SumDenOutMin=[]  SumDenOutMax=[]  SumNumOutMin=[]  SumNumOutMax=[]  DivideOutMin=[]  DivideOutMax=[]  IntegratorContinuousStateAttributes=''  IntegratorStateMustResolveToSignalObject=off  IntegratorRTWStateStorageClass=Auto  FilterContinuousStateAttributes=''  FilterStateMustResolveToSignalObject=off  FilterRTWStateStorageClass=Auto  ParallelPVariant=InternalParameters  IdealPVariant=Disabled  IVariant=InternalParameters  DVariant=InternalParameters  IntegratorVariant=Continuous  SatVariant=Disabled  AWVariant=Passthrough  PCopyVariant=Disabled  TRVariant=Disabled  FdbkBlocksVariant=Forward  IdealPFdbkVariant=Disabled  SatFdbkVariant=Disabled  DerivativeFilterVariant=ContFilter  NVariant=InternalParameters  NCopyVariant=Disabled  FilterICVariant=InternalICsFilter  IntegratorICVariant=InternalICs  ExternalResetVariant=Disabled  TRSumVariant=Passthrough  SumFdbkVariant=Disabled  SumVariant=Sum_PID
  SMC_LKA_controler : Subsystem
  Terminator : Terminator
  Terminator1 : Terminator
  signal processing : Subsystem
  steering_angle : Outport  VectorParamsAs1DForOutWhenUnconnected=off
  wires:
  SMC_LKA_controler/1(Out2) -> Terminator1/1
  signal processing/1(offset_at_prviewtime1) -> ?
  signal processing/2(qulv_at_prviewtime2) -> Multiport Switch2/3
  Constant/1 -> Multiport Switch/2
  [LKA_Main] -> Multiport Switch/1
  Multiport Switch/1 -> steering_angle/1  "STA"
  Constant1/1 -> Multiport Switch1/2
  [LKA_Main] -> Multiport Switch1/1
  Multiport Switch1/1 -> PID Controller/1  "OFST_PRV"
  Constant2/1 -> Multiport Switch2/2
  [LKA_Main] -> Multiport Switch2/1
  Multiport Switch2/1 -> Terminator/1  "CRUV_PRV"
  PID Controller/1 -> Multiport Switch/3
  [deviation_from_prescan] -> Multiport Switch1/3

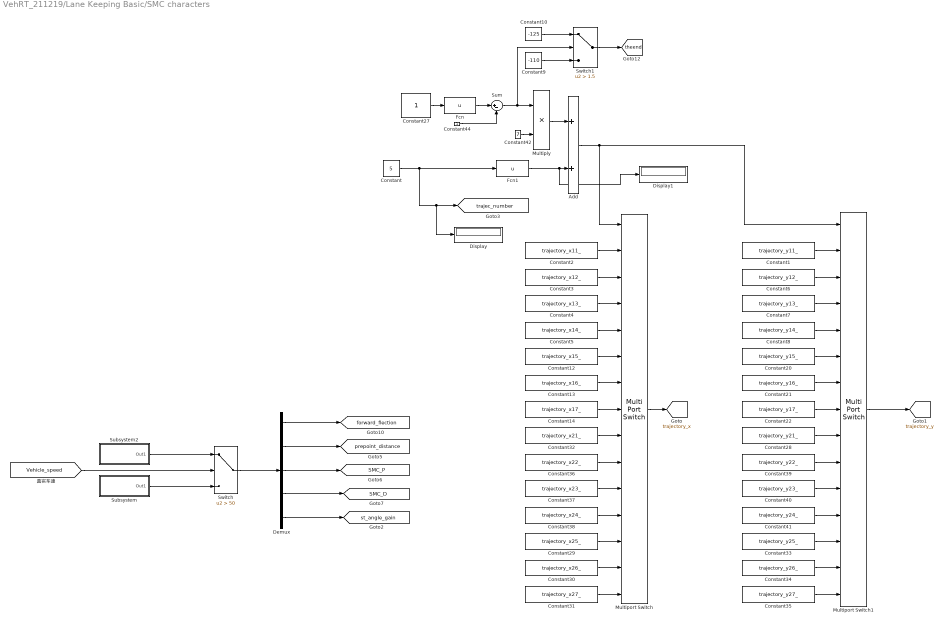
== system VehRT_211219/Lane Keeping Basic/SMC characters ==
  Add : Sum
  Constant : Constant  Value=5
  Constant1 : Constant  Value=trajectory_y11_
  Constant10 : Constant  Value=-125
  Constant12 : Constant  Value=trajectory_x15_
  Constant13 : Constant  Value=trajectory_x16_
  Constant14 : Constant  Value=trajectory_x17_
  Constant2 : Constant  Value=trajectory_x11_
  Constant20 : Constant  Value=trajectory_y15_
  Constant21 : Constant  Value=trajectory_y16_
  Constant22 : Constant  Value=trajectory_y17_
  Constant27 : Constant
  Constant28 : Constant  Value=trajectory_y21_
  Constant29 : Constant  Value=trajectory_x25_
  Constant3 : Constant  Value=trajectory_x12_
  Constant30 : Constant  Value=trajectory_x26_
  Constant31 : Constant  Value=trajectory_x27_
  Constant32 : Constant  Value=trajectory_x21_
  Constant33 : Constant  Value=trajectory_y25_
  Constant34 : Constant  Value=trajectory_y26_
  Constant35 : Constant  Value=trajectory_y27_
  Constant36 : Constant  Value=trajectory_x22_
  Constant37 : Constant  Value=trajectory_x23_
  Constant38 : Constant  Value=trajectory_x24_
  Constant39 : Constant  Value=trajectory_y22_
  Constant4 : Constant  Value=trajectory_x13_
  Constant40 : Constant  Value=trajectory_y23_
  Constant41 : Constant  Value=trajectory_y24_
  Constant42 : Constant  Value=7
  Constant44 : Constant
  Constant5 : Constant  Value=trajectory_x14_
  Constant6 : Constant  Value=trajectory_y12_
  Constant7 : Constant  Value=trajectory_y13_
  Constant8 : Constant  Value=trajectory_y14_
  Constant9 : Constant  Value=-110
  Demux : Demux  Outputs=5
  Display : Display
  Display1 : Display
  Fcn : Fcn  Expr=u
  Fcn1 : Fcn  Expr=u
  Multiply : Product
  Multiport Switch : MultiPortSwitch  Inputs=14  AllowDiffInputSizes=on
  Multiport Switch1 : MultiPortSwitch  Inputs=14  AllowDiffInputSizes=on
  Subsystem : Subsystem
  Subsystem2 : Subsystem
  Sum : Sum  Inputs=|+-
  Switch : Switch  Criteria=u2 > Threshold  Threshold=50
  Switch1 : Switch  Criteria=u2 > Threshold  Threshold=1.5
  tag scope: SMC_D=global, SMC_P=global, forward_flection=global, prepoint_distance=global, st_angle_gain=global, theend=global, trajec_number=global, trajectory_x=global, trajectory_y=global
  wires:
  Constant1/1 -> Multiport Switch1/2
  Constant2/1 -> Multiport Switch/2
  Constant3/1 -> Multiport Switch/3
  Constant4/1 -> Multiport Switch/4
  Constant5/1 -> Multiport Switch/5
  Constant6/1 -> Multiport Switch1/3
  Constant7/1 -> Multiport Switch1/4
  Constant8/1 -> Multiport Switch1/5
  Multiport Switch/1 -> [trajectory_x]
  Multiport Switch1/1 -> [trajectory_y]
  Constant12/1 -> Multiport Switch/6
  Constant13/1 -> Multiport Switch/7
  Constant14/1 -> Multiport Switch/8
  Constant22/1 -> Multiport Switch1/8
  Constant21/1 -> Multiport Switch1/7
  Constant20/1 -> Multiport Switch1/6
  Constant29/1 -> Multiport Switch/13
  Constant37/1 -> Multiport Switch/11
  Constant31/1 -> Multiport Switch/15
  Constant38/1 -> Multiport Switch/12
  Constant32/1 -> Multiport Switch/9
  Constant36/1 -> Multiport Switch/10
  Constant30/1 -> Multiport Switch/14
  Constant40/1 -> Multiport Switch1/11
  Constant35/1 -> Multiport Switch1/15
  Constant41/1 -> Multiport Switch1/12
  Constant39/1 -> Multiport Switch1/10
  Constant34/1 -> Multiport Switch1/14
  Constant28/1 -> Multiport Switch1/9
  Constant33/1 -> Multiport Switch1/13
  Constant27/1 -> Fcn/1
  Constant42/1 -> Multiply/2
  Sum/1 -> Switch1/2, Multiply/1
  Constant44/1 -> Sum/2
  Multiply/1 -> Add/1
  Constant/1 -> Display/1, [trajec_number], Fcn1/1
  Add/1 -> Multiport Switch1/1, Multiport Switch/1
  Switch/1 -> Demux/1
  Subsystem/1(Out1) -> Switch/3
  [Vehicle_speed] -> Switch/2
  Subsystem2/1(Out1) -> Switch/1
  Demux/4 -> [SMC_D]
  Demux/5 -> [st_angle_gain]
  Demux/3 -> [SMC_P]
  Demux/2 -> [prepoint_distance]
  Demux/1 -> [forward_flection]
  Constant10/1 -> Switch1/1
  Constant9/1 -> Switch1/3
  Switch1/1 -> [theend]
  Fcn/1 -> Sum/1
  Fcn1/1 -> Display1/1, Add/2
